simulink model "Stau_2Zellen"  (R2021a)
settings: Solver=VariableStepAuto  StartTime=0.0  StopTime=1  RelTol=1e-3
model workspace (MAT data in the model file):
  Kz = Simulink.Parameter
  Kz.Value = Simulink.data.Expression
  Kz.Value.ExpressionString = "(L/(Lc+ds))"
  Kz.DataType = 'auto'
  Kz.Dimensions = -1
  L = Simulink.Parameter
  L.Value = 52.8
  L.DataType = 'auto'
  L.Dimensions = [1 1]
  Lc = Simulink.Parameter
  Lc.Value = 4.4
  Lc.DataType = 'auto'
  Lc.Dimensions = [1 1]
  Rk = Simulink.Parameter
  Rk.Value = Simulink.data.Expression
  Rk.Value.ExpressionString = "Lc/v"
  Rk.DataType = 'auto'
  Rk.Dimensions = -1
  Tz = Simulink.Parameter
  Tz.Value = Simulink.data.Expression
  Tz.Value.ExpressionString = "L/v"
  Tz.DataType = 'auto'
  Tz.Dimensions = -1
  ds = Simulink.Parameter
  ds.Value = Simulink.data.Expression
  ds.Value.ExpressionString = "dt*v"
  ds.DataType = 'auto'
  ds.Dimensions = -1
  dt = Simulink.Parameter
  dt.Value = 1
  dt.DataType = 'auto'
  dt.Dimensions = [1 1]
  v = Simulink.Parameter
  v.Value = 13.89
  v.DataType = 'auto'
  v.Dimensions = [1 1]
libraries: EdgesLibrary x3, StreetLanesLibrary x2
settings Model: OrderedModelArguments=off  Creator=phill  LastModifiedBy=timyb
settings SolverCC: ZeroCrossAlgorithm=Adaptive

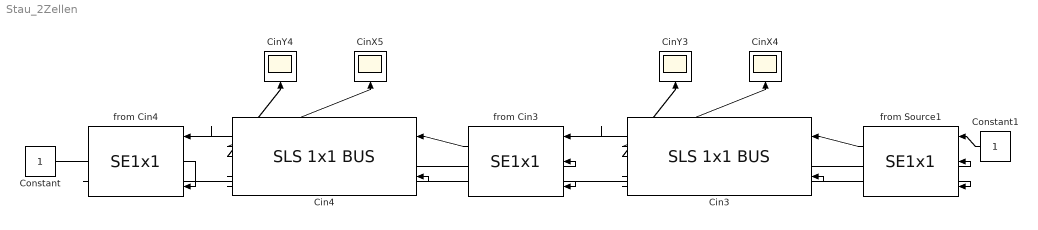
== system Stau_2Zellen ==
  Cin3 : StreetLanesLibrary/SLS 1x1 BUS  Kz=1  Tz=1
  Cin4 : StreetLanesLibrary/SLS 1x1 BUS  Kz=1  Tz=1
  CinX4 : Scope
  CinX5 : Scope
  CinY3 : Scope
  CinY4 : Scope
  Constant : Constant
  Constant1 : Constant
  from Cin3 : EdgesLibrary/SE1x1  Rk=1
  from Cin4 : EdgesLibrary/SE1x1  Rk=1
  from Source1 : EdgesLibrary/SE1x1  Rk=1
  wires:
  from Source1/1 -> Cin3/1
  Cin3/6 -> from Source1/2
  Cin4/2 -> from Cin4/1
  Cin4/7 -> from Cin3/3
  Cin3/2 -> from Cin3/1
  from Cin3/1 -> Cin4/1
  from Cin3/2 -> Cin3/2
  Cin4/6 -> from Cin3/2
  Cin4/4 -> CinY4/1
  Cin3/7 -> from Source1/3
  from Cin4/2 -> Cin4/2
  Cin3/3 -> CinX4/1
  Cin3/4 -> CinY3/1
  Cin4/3 -> CinX5/1
  Constant/1 -> from Cin4/3
  Constant1/1 -> from Source1/1
